simulink model "nid_cvst_kinect_sdk_sensor_angle"  (Simulink 7.6)
settings: Solver=FixedStepDiscrete  StartTime=0.0  StopTime=inf  RelTol=1e-3
libraries: vipsnks x2, nid_lib x2, simulink x1
settings Model: Creator=tchikama  LastModifiedBy=tchikama
settings DataIOCC: SaveOutput=off
settings OptimizationCC: SimCompilerOptimization=On
settings HardwareCC: ProdIntDivRoundTo=Zero  ProdEndianess=LittleEndian  ProdHWDeviceType=Generic->32-bit x86 compatible
settings RTWCC: ProcessScript=grt_make_rtw_hook  RTWCompilerOptimization=On
settings CodeAppCC: MaxIdLength=95

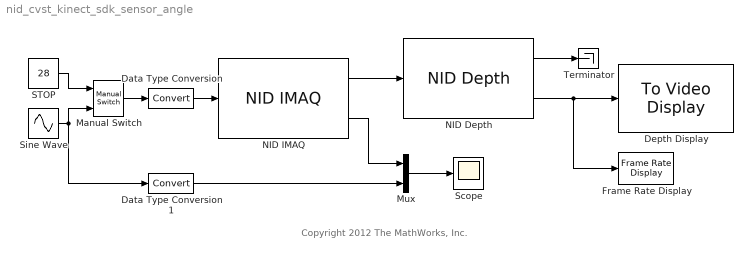
== system nid_cvst_kinect_sdk_sensor_angle ==
  note: Copyright 2012 The MathWorks, Inc.
  Data Type Conversion : DataTypeConversion
  Data Type Conversion1 : DataTypeConversion
  Depth Display : vipsnks/To Video Display  DialogControllerArgs=DataTag0  inputType=Obsolete  imagePorts=One multidimensional signal  OutputDevice=On-screen video monitor  fullScreen=off  videoWindowX=872  videoWindowY=173  saveWindowSize=off  videoWindowWidth=640  videoWindowHeight=480  dataOrg=Column-major  openAtMdlStart=on  isWindowOpen=on
  Frame Rate Display : vipsnks/Frame Rate Display  DialogController=vipDDGCreate  DialogControllerArgs=DataTag1  UpdateRate=10
  Manual Switch : simulink/Signal Routing/Manual Switch  SystemSampleTime=-1  sw=0  action=0  varsize=off
  Mux : Mux  Inputs=2
  NID Depth : nid_lib/NID Depth  depthOutput=Depth  conv_XYZ_RW=off  viewer=on
  NID IMAQ : nid_lib/NID IMAQ  imaq_depth=on  imaq_motion=off  imaq_image=off  view_point=off  imaq_skeleton=off  imaq_ir=off  mirror_image=off  imaq_sample_time=1/30  res_fps=VGA (640x480): 30 FPS  needPsiPose=off  angle_input=on  angle=0  angle_read=on  near_mode=off  seated_mode=off
  STOP : Constant  Value=28
  Scope : Scope
      settings: TimeRange=30  YMin=-20  YMax=20
  Sine Wave : Sin  SineType=Sample based  Amplitude=20  Samples=900  SampleTime=1/30
  Terminator : Terminator
  wires:
  NID IMAQ/1 -> NID Depth/1
  NID Depth/2 -> Depth Display/1, Frame Rate Display/1
  NID Depth/1 -> Terminator/1
  Mux/1 -> Scope/1
  NID IMAQ/2 -> Mux/1
  Data Type Conversion/1 -> NID IMAQ/1
  Manual Switch/1 -> Data Type Conversion/1
  STOP/1 -> Manual Switch/1
  Sine Wave/1 -> Manual Switch/2, Data Type Conversion1/1
  Data Type Conversion1/1 -> Mux/2
